simulink model "bit4counter"  (R2020a)
settings: Solver=VariableStepAuto  StartTime=0.0  StopTime=10.0  RelTol=1e-3
libraries: simulink_extras x4
settings Model: Creator=kishan  LastModifiedBy=kishan

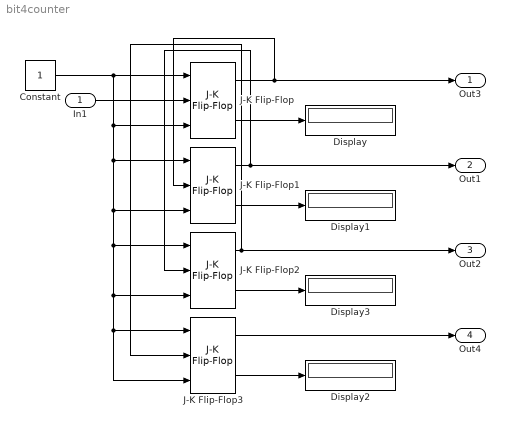
== system bit4counter ==
  In1 : Inport
  Constant : Constant
  Display{,1..3} (4 alike) : Display
  J-K Flip-Flop{,1..3} (4 alike) : simulink_extras/Flip Flops/J-K Flip-Flop  initial_condition=0
  Out3 : Outport
  Out1 : Outport  Port=2
  Out2 : Outport  Port=3
  Out4 : Outport  Port=4
  wires:
  J-K Flip-Flop3/1 -> Out4/1
  J-K Flip-Flop1/1 -> Out1/1, J-K Flip-Flop2/2
  J-K Flip-Flop2/1 -> Out2/1, J-K Flip-Flop3/2
  J-K Flip-Flop/1 -> Out3/1, J-K Flip-Flop1/2
  In1/1 -> J-K Flip-Flop/2
  Constant/1 -> J-K Flip-Flop2/1, J-K Flip-Flop3/1, J-K Flip-Flop3/3, J-K Flip-Flop2/3, J-K Flip-Flop1/3, J-K Flip-Flop1/1, J-K Flip-Flop/3, J-K Flip-Flop/1
  J-K Flip-Flop/2 -> Display/1
  J-K Flip-Flop1/2 -> Display1/1
  J-K Flip-Flop3/2 -> Display2/1
  J-K Flip-Flop2/2 -> Display3/1
